simulink model "received_OK_backup"  (R2015b)
settings: Solver=VariableStepAuto  StartTime=0.0  StopTime=10.0  RelTol=1e-3
settings Model: Creator=Administrator  LastModifiedBy=Administrator

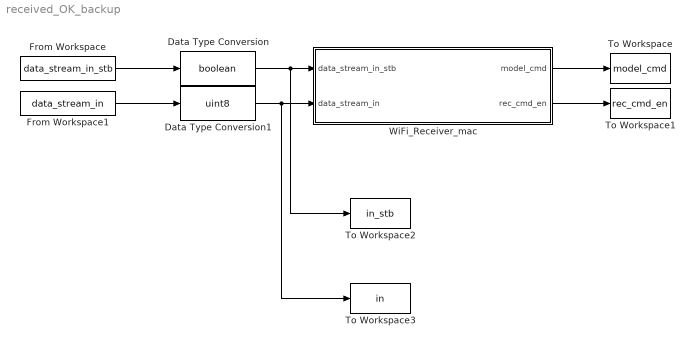
== system received_OK_backup ==
  Data Type Conversion : DataTypeConversion  OutDataTypeStr=boolean
  Data Type Conversion1 : DataTypeConversion  OutDataTypeStr=uint8
  From Workspace : FromWorkspace  VariableName=data_stream_in_stb  OutDataTypeStr=double  SampleTime=0
  From Workspace1 : FromWorkspace  VariableName=data_stream_in  OutDataTypeStr=double  SampleTime=0
  To Workspace : ToWorkspace  VariableName=model_cmd  SaveFormat=Timeseries  SampleTime=-1
  To Workspace1 : ToWorkspace  VariableName=rec_cmd_en  SaveFormat=Timeseries  SampleTime=-1
  To Workspace2 : ToWorkspace  VariableName=in_stb  SaveFormat=Timeseries  SampleTime=-1
  To Workspace3 : ToWorkspace  VariableName=in  SaveFormat=Timeseries  SampleTime=-1
  WiFi_Receiver_mac : Stateflow chart  TreatAsAtomicUnit=on
  wires:
  Data Type Conversion/1 -> To Workspace2/1, WiFi_Receiver_mac/1(data_stream_in_stb)
  From Workspace/1 -> Data Type Conversion/1
  From Workspace1/1 -> Data Type Conversion1/1
  WiFi_Receiver_mac/1(model_cmd) -> To Workspace/1
  WiFi_Receiver_mac/2(rec_cmd_en) -> To Workspace1/1
  Data Type Conversion1/1 -> To Workspace3/1, WiFi_Receiver_mac/2(data_stream_in)

== stateflow chart received_OK_backup/WiFi_Receiver_mac ==
  settings: executeAtInitialization=1
  state wait_cmd
    entry:
    model_cmd=0;
    rec_cmd_en=0;
  state initial
    entry:
    model_cmd=0;
    rec_cmd_en=0;
    time_cnt=0;
  state received_OK
    entry:
    model_cmd=1;
    rec_cmd_en=1;
  state detect_cmd
  state received_O
  state received_K
  state received_ERROR
    entry:
    model_cmd=2;
    rec_cmd_en=1;
  state time_out
    time_cnt=0;
    model_cmd=2;
    rec_cmd_en=1;
  state received_E
  state received_R
  state received_R1
  state received_O1
  state received_R2
  state received_FAIL
    entry:
    model_cmd=3;
    rec_cmd_en=1;
  state received_F
  state received_A
  state received_I
  state received_L
  (junction 129) -> wait_cmd
  (junction 13) -> (junction 129) [order 2] : [data_stream_in~=75]
  (junction 22) -> wait_cmd : [(data_stream_in~=79)&&(data_stream_in~=69)&&(data_stream_in~=70)]
  (junction 18) -> (junction 22) [order 2]
  (default) -> initial
  (junction 10) -> received_O [order 1] : [data_stream_in_stb==0]
  received_OK -> detect_cmd
  received_K -> received_OK
  wait_cmd -> (junction 6)
  (junction 6) -> (junction 18) : [data_stream_in_stb==1]
  (junction 18) -> received_O [order 1] : [data_stream_in==79]
  received_O -> (junction 10)
  (junction 10) -> (junction 13) [order 2] : [data_stream_in_stb==1]
  (junction 13) -> received_K [order 1] : [data_stream_in==75]
  initial -> wait_cmd
  (junction 18) -> (junction 38) [order 3] : [data_stream_in_stb==0]{time_cnt = time_cnt + 1;}
  (junction 38) -> wait_cmd [order 2] : [time_cnt<=60000000]
  (junction 38) -> time_out [order 1] : [time_cnt>60000000]
  (junction 38) -> (junction 52) [order 3]
  (junction 79) -> received_O1 [order 2] : [data_stream_in_stb==0]
  (junction 73) -> received_R1 [order 2] : [data_stream_in_stb==0]
  (junction 55) -> received_E [order 1] : [data_stream_in_stb==0]
  (junction 66) -> received_R [order 2] : [data_stream_in_stb==0]
  received_ERROR -> detect_cmd
  received_R2 -> received_ERROR
  received_E -> (junction 55)
  (junction 55) -> (junction 56) [order 2] : [data_stream_in_stb==1]
  (junction 56) -> received_R [order 1] : [data_stream_in==82]
  received_R -> (junction 66)
  (junction 66) -> (junction 64) [order 1] : [data_stream_in_stb==1]
  (junction 64) -> received_R1 [order 1] : [data_stream_in==82]
  received_R1 -> (junction 73)
  (junction 73) -> (junction 71) [order 1] : [data_stream_in_stb==1]
  (junction 71) -> received_O1 [order 1] : [data_stream_in==79]
  received_O1 -> (junction 79)
  (junction 79) -> (junction 77) [order 1] : [data_stream_in_stb==1]
  (junction 77) -> received_R2 [order 1] : [data_stream_in==82]
  (junction 52) -> received_E [order 1] : [data_stream_in==69]
  (junction 77) -> (junction 132) [order 2] : [data_stream_in~=82]
  (junction 71) -> (junction 132) [order 2] : [data_stream_in~=79]
  (junction 64) -> (junction 132) [order 2] : [data_stream_in~=82]
  time_out -> wait_cmd
  (junction 52) -> (junction 124) [order 2]
  (junction 56) -> (junction 132) [order 2] : [data_stream_in~=82]
  (junction 132) -> wait_cmd
  (junction 97) -> received_I [order 2] : [data_stream_in_stb==0]
  (junction 123) -> received_F [order 1] : [data_stream_in_stb==0]
  (junction 121) -> received_A [order 2] : [data_stream_in_stb==0]
  received_L -> received_FAIL
  (junction 124) -> received_F : [data_stream_in==70]
  received_F -> (junction 123)
  (junction 123) -> (junction 114) [order 2] : [data_stream_in_stb==1]
  (junction 114) -> received_A [order 1] : [data_stream_in==65]
  received_A -> (junction 121)
  (junction 121) -> (junction 119) [order 1] : [data_stream_in_stb==1]
  (junction 119) -> received_I [order 1] : [data_stream_in==73]
  received_I -> (junction 97)
  (junction 97) -> (junction 99) [order 1] : [data_stream_in_stb==1]
  (junction 99) -> received_L [order 1] : [data_stream_in==76]
  received_FAIL -> detect_cmd
  (junction 99) -> (junction 138) [order 2] : [data_stream_in~=76]
  (junction 119) -> (junction 138) [order 2] : [data_stream_in~=73]
  (junction 114) -> (junction 138) [order 2] : [data_stream_in~=65]
  (junction 138) -> wait_cmd
  detect_cmd -> (junction 32)
  (junction 34) -> wait_cmd
  (junction 32) -> (junction 34)
  data: data_stream_in_stb input boolean; data_stream_in input uint8; model_cmd output fixdt(0,4,0); rec_cmd_en output boolean; time_cnt local double
